simulink model "Corpo_Borboleta"  (R2025b)
settings: Solver=VariableStepAuto  StartTime=0.0  StopTime=10.0  RelTol=1e-3
undefined symbols (not defined in the file): cd, kappa, R
settings Model: Creator=ivomu  LastModifiedBy=ivomu

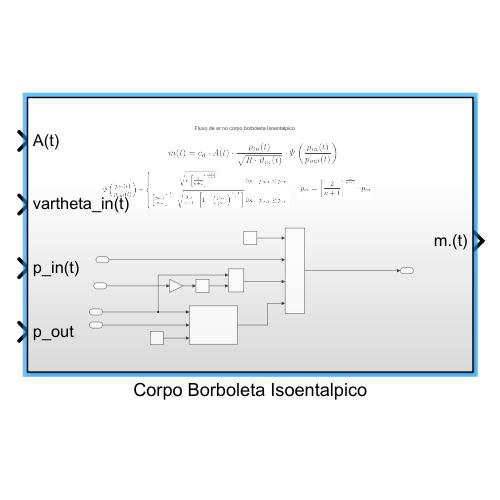
[thumbnail: Simulink's stored preview of the top-level diagram]
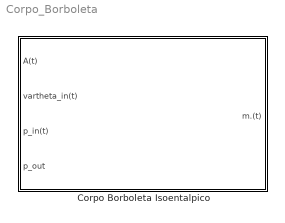
== system Corpo_Borboleta ==
  Corpo Borboleta Isoentalpico : Subsystem

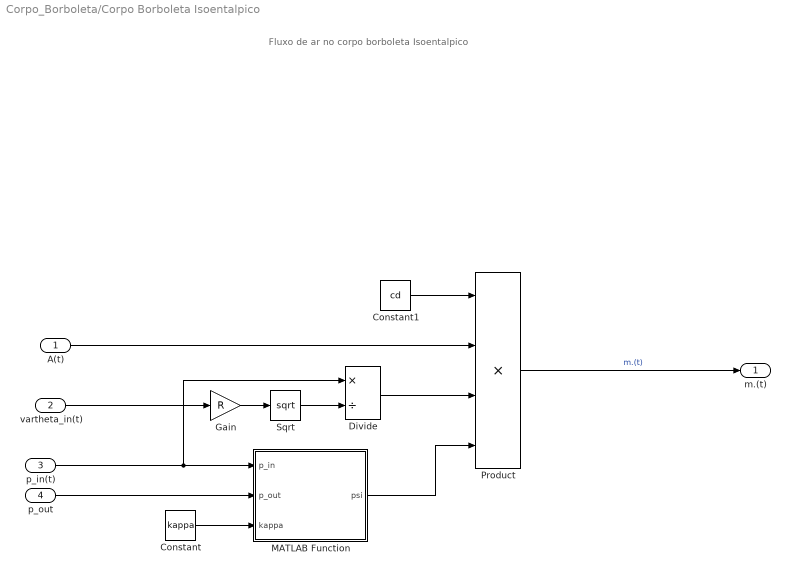
== system Corpo_Borboleta/Corpo Borboleta Isoentalpico ==
  note: Fluxo de ar no corpo borboleta Isoentalpico
  A(t) : Inport
  vartheta_in(t) : Inport  Port=2
  p_in(t) : Inport  Port=3
  p_out : Inport  Port=4
  Constant : Constant  Value=kappa
  Constant1 : Constant  Value=cd
  Divide : Product  Inputs=*/
  Gain : Gain  Gain=R
  MATLAB Function : MATLAB Function  TreatAsAtomicUnit=on
  Product : Product  Inputs=4
  Sqrt : Sqrt
  m.(t) : Outport
  wires:
  Constant/1 -> MATLAB Function/3(kappa)
  MATLAB Function/1(psi) -> Product/4
  p_in(t)/1 -> Divide/1, MATLAB Function/1(p_in)
  Sqrt/1 -> Divide/2
  Gain/1 -> Sqrt/1
  Divide/1 -> Product/3
  Constant1/1 -> Product/1
  Product/1 -> m.(t)/1  "m.(t)"
  A(t)/1 -> Product/2
  vartheta_in(t)/1 -> Gain/1
  p_out/1 -> MATLAB Function/2(p_out)

== matlab function Corpo_Borboleta/Corpo Borboleta Isoentalpico/MATLAB Function ==
  data: p_in input; psi output; p_out input; kappa input
function psi = psiFcn(p_in, p_out, kappa)
%psiFcn Função de fluxo Ψ
%   Detailed explanation goes here
arguments (Input)
    p_in;       %pressão de entrada
    p_out;      %pressão de saida;
    kappa;
end

arguments (Output)
    psi
end
    p_cr = p_in * (2/(kappa+1))^(kappa/(kappa-1));
    if p_out < p_cr
        % Fluxo Sônico (Choked)
        psi = sqrt(kappa * (2/(kappa+1))^((kappa+1)/(kappa-1)));
    else
        % Fluxo Subsônico
        term1 = (p_out/p_in)^(1/kappa);
        term2 = sqrt((2*kappa)/(kappa-1) * (1 - (p_out/p_in)^((kappa-1)/kappa)));
        psi = term1 * term2;
    end
end
